simulink model "FilterRealization"  (R2019b)
settings: Solver=VariableStepAuto  StartTime=0.0  StopTime=10.0  RelTol=1e-3
settings Model: Creator=ip  LastModifiedBy=ip

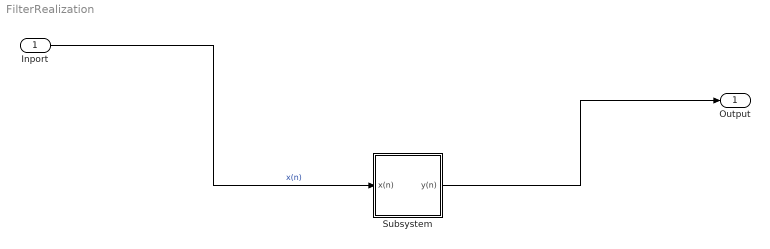
== system FilterRealization ==
  Inport : Inport
  Subsystem : Subsystem
  Output : Outport
  wires:
  Inport/1 -> Subsystem/1(x(n))  "x(n)"
  Subsystem/1(y(n)) -> Output/1

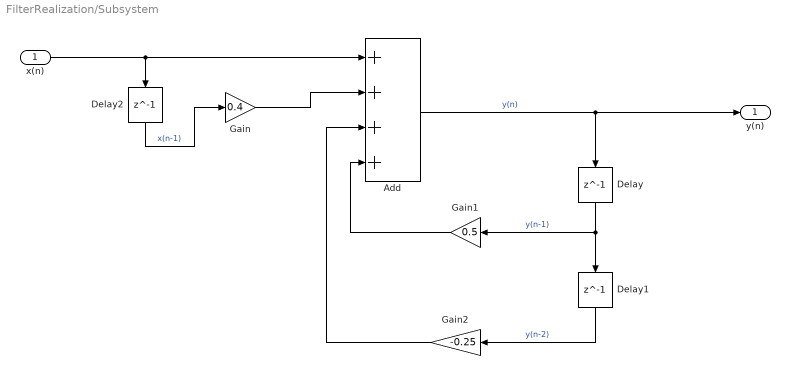
== system FilterRealization/Subsystem ==
  x(n) : Inport
  Add : Sum  Inputs=4
  Delay : Delay  DelayLength=1
  Delay1 : Delay  DelayLength=1
  Delay2 : Delay  DelayLength=1
  Gain : Gain  Gain=0.4
  Gain1 : Gain  Gain=0.5
  Gain2 : Gain  Gain=-0.25
  y(n) : Outport
  wires:
  Gain2/1 -> Add/3
  Delay2/1 -> Gain/1  "x(n-1)"
  Delay/1 -> Gain1/1, Delay1/1  "y(n-1)"
  Gain/1 -> Add/2
  Delay1/1 -> Gain2/1  "y(n-2)"
  Gain1/1 -> Add/4
  Add/1 -> y(n)/1, Delay/1  "y(n)"
  x(n)/1 -> Add/1, Delay2/1
